simulink model "MARCH_v1_2"  (R2016a)
settings: Solver=FixedStepDiscrete  StartTime=0.0  StopTime=10  FixedStep=.001  RelTol=1e-3
PreLoadFcn:
  | load db.mat
  | initialize_model_param
PostLoadFcn:
  | build_location = fullfile(fileparts(which(bdroot)),'build');
  | 
  | set_param(0, 'CacheFolder', build_location);
  | set_param(0, 'CodeGenFolder', build_location);
InitFcn:
  | % Change dir to model location
  | cd(fileparts(which(bdroot)));
  | 
  | % Run init script
  | init_model;
StartFcn:
  | % Make sure we always move back to model folder
  | cd(fileparts(which(bdroot)));
StopFcn:
  | % Make sure we always move back to model folder
  | cd(fileparts(which(bdroot)));
values from neighbouring files (symbols this model uses):
  n = 1000    [initialize_model_param.m]
undefined symbols (not defined in the file or in its folder): par
libraries: xpcethercatlib x21, slrtlib x5
CloseFcn:
  | % Make sure we always move back to model folder
  | cd(fileparts(which(bdroot)));
  | 
  | set_param(0, 'CacheFolder', '');
  | set_param(0, 'CodeGenFolder', '');
PauseFcn:
  | % Make sure we always move back to model folder
  | cd(fileparts(which(bdroot)));
ContinueFcn:
  | % Make sure we always move back to model folder
  | cd(fileparts(which(bdroot)));
settings Model: SimulationMode=external  Creator=rtheyyun  LastModifiedBy=Projectmarch
settings SolverCC: EnableConcurrentExecution=on  ConcurrentTasks=on
settings DataIOCC: LimitDataPoints=on  SaveFinalState=on  SaveFormat=StructureWithTime  SignalLoggingSaveFormat=ModelDataLogs  InspectSignalLogs=on
settings OptimizationCC: BlockReduction=off  OptimizeBlockIOStorage=off  BufferReuse=off  GlobalBufferReuse=off  ExpressionFolding=off  ExpressionDepthLimit=2147483647  LocalBlockOutputs=off
settings DebuggingCC: ReadBeforeWriteMsg=DisableAll  WriteAfterWriteMsg=DisableAll  WriteAfterReadMsg=DisableAll  UnderspecifiedInitializationDetection=Classic  MergeDetectMultiDrivingBlocksExec=none  SolverPrmCheckMsg=warning  InheritedTsInSrcMsg=none  FcnCallInpInsideContextMsg=UseLocalSettings  AllowSymbolicDim=off  StateNameClashWarn=warning
settings HardwareCC: ProdBitPerPointer=32  ProdLargestAtomicFloat=None  ProdWordSize=32  ProdLongLongMode=on  ProdHWDeviceType=Generic->32-bit x86 compatible
settings ModelReferenceCC: UpdateModelReferenceTargets=Force  PropagateSignalLabelsOutOfModel=off
settings RTWCC: SystemTargetFile=slrt.tlc  TemplateMakefile=slrt_default_tmf  Description=Simulink Real-Time  RTWVerbose=off  RTWCompilerOptimization=on
settings SimulinkRealTimeCC: GeneratePreprocessorConditionals=Disable all  xPCisModelTimeout=off  xPCModelTimeoutSecs=20  xPCConcurrentTasks=on
settings ConfigComp: CovModelRefEnable=Off  CovSFcnEnable=off

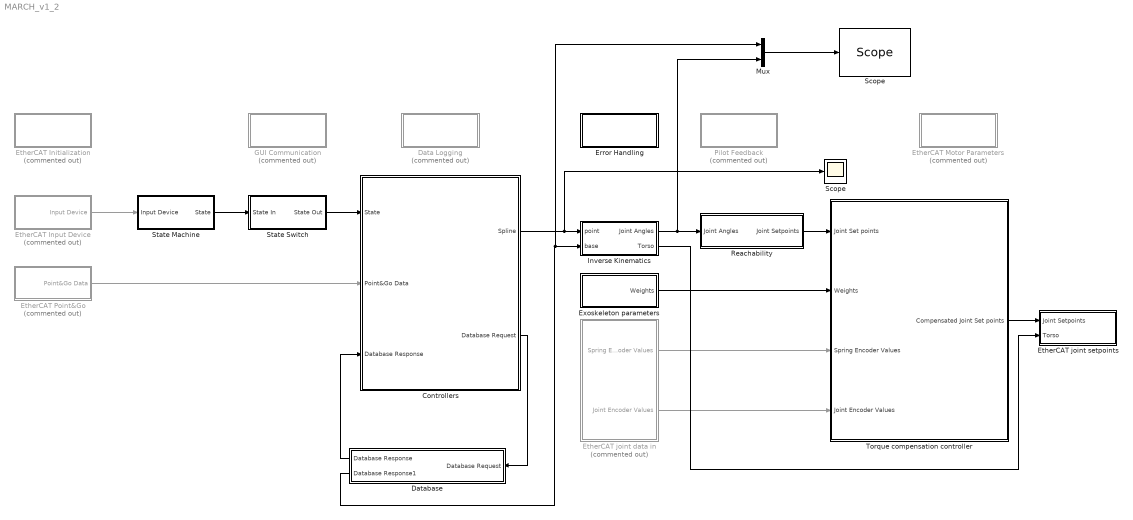
== system MARCH_v1_2 ==
  Controllers : Subsystem
  Data Logging : Subsystem  Commented=on
  Database : Subsystem
  Error Handling : Subsystem
  EtherCAT Initialization : Subsystem  Commented=on
  EtherCAT Input Device : Subsystem  Commented=on
  EtherCAT Motor Parameters : Subsystem  Commented=on
  EtherCAT Point&Go : Subsystem  Commented=on
  EtherCAT joint data in : Subsystem  Commented=on
  EtherCAT joint setpoints : Subsystem
  Exoskeleton parameters : Subsystem
  GUI Communication : Subsystem  Commented=on
  Inverse Kinematics : Subsystem
  Mux : Mux  Inputs=2
  Pilot Feedback : Subsystem  Commented=on
  Reachability : Subsystem
  Scope : Scope
  "Scope " : slrtlib/Displays and Logging/Scope   scopeno=2  scopetype=Target  autostart=on  viewmode=Graphical rolling  formatstr='%15.6f'  grid=on  ylimits=[0,0]  nosamples=25000  noprepostsamples=0  interleave=1  triggermode=FreeRun  triggersignal=1  trigsignalfromport=off  triggerlevel=0.0  triggerslope=Either  triggerscope=1  triggersample=0  filename=data.dat  mode=Lazy  writesize=512  autorestart=off  dynamicfilemode=off  maxwritefilesize=512*1024^2
  State Machine : Subsystem
  State Switch : Subsystem
  Torque compensation controller : Subsystem
  wires:
  Torque compensation controller/1(Compensated Joint Set points) -> EtherCAT joint setpoints/1(Joint Setpoints)
  Reachability/1(Joint Setpoints) -> Torque compensation controller/1(Joint Set points)
  Inverse Kinematics/1(Joint Angles) -> Mux/2, Reachability/1(Joint Angles)
  State Switch/1(State Out) -> Controllers/1(State)
  Controllers/1(Spline) -> Scope/1, Inverse Kinematics/1(point)
  State Machine/1(State) -> State Switch/1(State In)
  Controllers/2(Database Request) -> Database/1(Database Request)
  Database/1(Database Response) -> Controllers/3(Database Response)
  EtherCAT joint data in/1(Spring Encoder Values) -> Torque compensation controller/3(Spring Encoder Values)
  EtherCAT joint data in/2(Joint Encoder Values) -> Torque compensation controller/4(Joint Encoder Values)
  Exoskeleton parameters/1(Weights) -> Torque compensation controller/2(Weights)
  EtherCAT Input Device/1(Input Device) -> State Machine/1(Input Device)
  EtherCAT Point&Go/1(Point&Go Data) -> Controllers/2(Point&Go Data)
  Mux/1 -> "Scope "/1
  Database/2(Database Response1) -> Mux/1, Inverse Kinematics/2(base)
  Inverse Kinematics/2(Torso) -> EtherCAT joint setpoints/2(Torso)

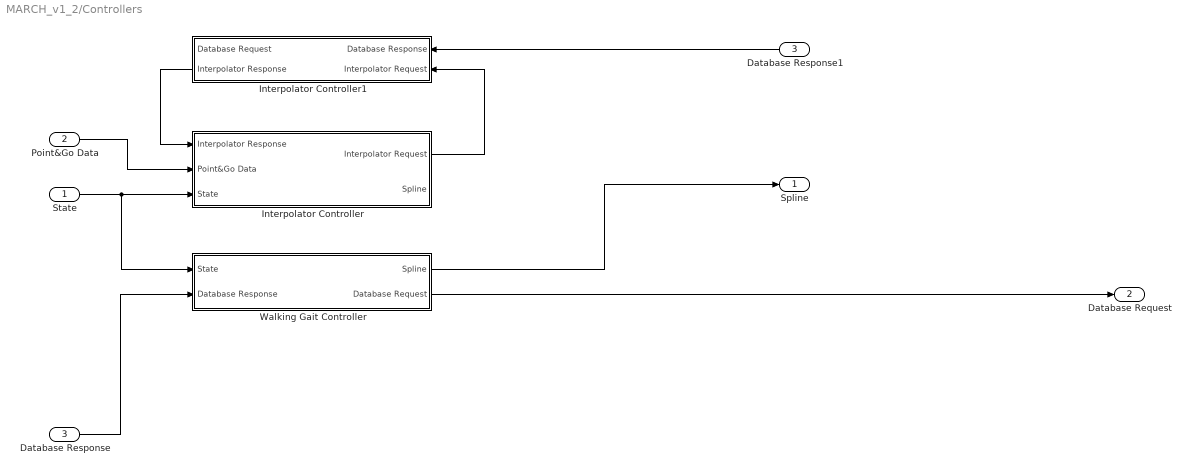
== system MARCH_v1_2/Controllers ==
  State : Inport
  Point&Go Data : Inport  Port=2
  Database Response : Inport  Port=3
  Database Response1 : InportShadow  Port=3
  Interpolator Controller : Subsystem
  Interpolator Controller1 : Subsystem
  Walking Gait Controller : Subsystem
  Spline : Outport
  Database Request : Outport  Port=2
  wires:
  State/1 -> Interpolator Controller/3(State), Walking Gait Controller/1(State)
  Database Response/1 -> Walking Gait Controller/2(Database Response)
  Interpolator Controller/1(Interpolator Request) -> Interpolator Controller1/2(Interpolator Request)
  Interpolator Controller1/2(Interpolator Response) -> Interpolator Controller/1(Interpolator Response)
  Database Response1/1 -> Interpolator Controller1/1(Database Response)
  Walking Gait Controller/2(Database Request) -> Database Request/1
  Walking Gait Controller/1(Spline) -> Spline/1
  Point&Go Data/1 -> Interpolator Controller/2(Point&Go Data)

== system MARCH_v1_2/Data Logging ==

== system MARCH_v1_2/Database ==
  Database Request : Inport
  Database Interface : MATLAB Function  TreatAsAtomicUnit=on
  Database Response : Outport
  Database Response1 : Outport  Port=2
  wires:
  Database Request/1 -> Database Interface/1(request)
  Database Interface/1(spline) -> Database Response/1
  Database Interface/2(swing) -> Database Response1/1

== system MARCH_v1_2/Error Handling ==

== system MARCH_v1_2/EtherCAT Initialization ==
  "EtherCAT Init " : xpcethercatlib/EtherCAT Init   Priority=0  config_file=D:\Software\MATLAB\simulink-models\EtherCAT Config files\quad_slave_both_legs_v1.0.xml  device_id=0  pci_bus=2  pci_slot=0  dctuning=0  enaDebug=off  enaDC=on  errLink=off  masterDbg=off  stateChgDbg=off  baseClock=off  masterCfg=off  logFile='c:\dbglog.txt'  sample_time=0.001000
  Terminator : Terminator
  wires:
  "EtherCAT Init "/1 -> Terminator/1

== system MARCH_v1_2/EtherCAT Input Device ==
  EtherCAT PDO Receive : xpcethercatlib/EtherCAT PDO Receive  Priority=2  sig_name=LHFE.Inputs.jointAngle  sig_offset=208  sig_type=uint32  type_size=32  sig_dim=1  device_id=0  sample_time=0.001000
  Input Device : Outport
  wires:
  EtherCAT PDO Receive/1 -> Input Device/1

== system MARCH_v1_2/EtherCAT Motor Parameters ==

== system MARCH_v1_2/EtherCAT Point&Go ==
  EtherCAT PDO Receive : xpcethercatlib/EtherCAT PDO Receive  Priority=2  sig_name=LHFE.Inputs.jointAngle  sig_offset=208  sig_type=uint32  type_size=32  sig_dim=1  device_id=0  sample_time=0.001000
  Point&Go Data : Outport
  wires:
  EtherCAT PDO Receive/1 -> Point&Go Data/1

== system MARCH_v1_2/EtherCAT joint data in ==
  Joint Encoder EtherCAT : Subsystem
  Spring Encoder EtherCAT : Subsystem  Commented=on
  Spring Encoder Values : Outport
  Joint Encoder Values : Outport  Port=2
  wires:
  Spring Encoder EtherCAT/1(Spring Encoder Values) -> Spring Encoder Values/1
  Joint Encoder EtherCAT/1(Joint Encoder Values) -> Joint Encoder Values/1

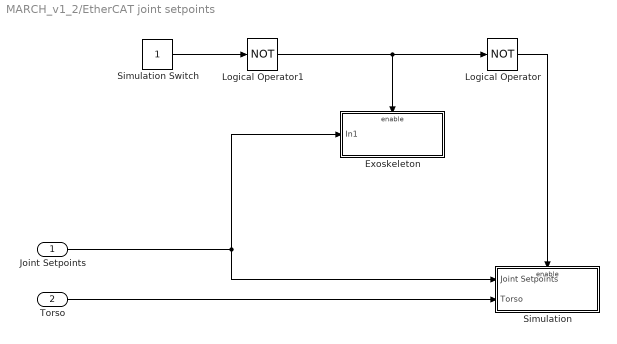
== system MARCH_v1_2/EtherCAT joint setpoints ==
  Joint Setpoints : Inport
  Torso : Inport  Port=2
  Exoskeleton : Subsystem  TreatAsAtomicUnit=on
  Logical Operator : Logic  Operator=NOT  AllPortsSameDT=off  OutDataTypeStr=boolean
  Logical Operator1 : Logic  Operator=NOT  AllPortsSameDT=off  OutDataTypeStr=boolean
  Simulation : Subsystem  TreatAsAtomicUnit=on
  Simulation Switch : Constant
  wires:
  Joint Setpoints/1 -> Exoskeleton/1(In1), Simulation/1(Joint Setpoints)
  Logical Operator1/1 -> Logical Operator/1, Exoskeleton/Enable
  Logical Operator/1 -> Simulation/Enable
  Simulation Switch/1 -> Logical Operator1/1
  Torso/1 -> Simulation/2(Torso)

== system MARCH_v1_2/Exoskeleton parameters ==
  Weights : Outport

== system MARCH_v1_2/GUI Communication ==

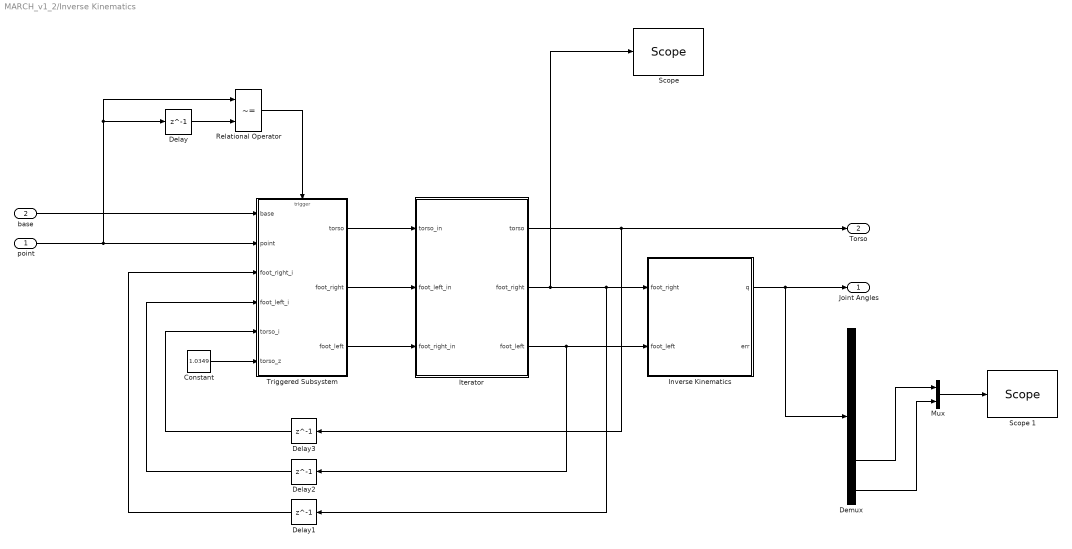
== system MARCH_v1_2/Inverse Kinematics ==
  point : Inport
  base : Inport  Port=2
  Constant : Constant  Value=1.0349
  Delay : Delay  DelayLength=1
  Delay1 : Delay  DelayLength=1  InitialCondition=[0.2073 -0.2467 -1.0349]
  Delay2 : Delay  DelayLength=1  InitialCondition=[0.2073 0.2467 -1.0349]
  Delay3 : Delay  DelayLength=1
  Demux : Demux  Outputs=6
  Inverse Kinematics : MATLAB Function  TreatAsAtomicUnit=on
  Iterator : MATLAB Function  TreatAsAtomicUnit=on
  Mux : Mux  Inputs=2
  Relational Operator : RelationalOperator  Operator=~=  OutDataTypeStr=boolean
  "Scope " : slrtlib/Displays and Logging/Scope   scopeno=1  scopetype=Target  autostart=on  viewmode=Numerical  formatstr='%15.6f'  grid=on  ylimits=[0,0]  nosamples=3  noprepostsamples=0  interleave=1  triggermode=FreeRun  triggersignal=1  trigsignalfromport=off  triggerlevel=0.0  triggerslope=Either  triggerscope=1  triggersample=0  filename=data.dat  mode=Lazy  writesize=512  autorestart=off  dynamicfilemode=off  maxwritefilesize=512*1024^2
  Scope 1 : slrtlib/Displays and Logging/Scope   scopeno=4  scopetype=Target  autostart=on  viewmode=Graphical sliding  formatstr='%15.6f'  grid=on  ylimits=[0,0]  nosamples=100  noprepostsamples=0  interleave=1  triggermode=FreeRun  triggersignal=1  trigsignalfromport=off  triggerlevel=0.0  triggerslope=Either  triggerscope=1  triggersample=0  filename=data.dat  mode=Lazy  writesize=512  autorestart=off  dynamicfilemode=off  maxwritefilesize=512*1024^2
  Triggered Subsystem : Subsystem  TreatAsAtomicUnit=on
  Joint Angles : Outport
  Torso : Outport  Port=2
  wires:
  Inverse Kinematics/1(q) -> Demux/1, Joint Angles/1
  Constant/1 -> Triggered Subsystem/6(torso_z)
  base/1 -> Triggered Subsystem/1(base)
  point/1 -> Relational Operator/1, Delay/1, Triggered Subsystem/2(point)
  Delay/1 -> Relational Operator/2
  Relational Operator/1 -> Triggered Subsystem/Trigger
  Triggered Subsystem/2(foot_right) -> Iterator/2(foot_left_in)
  Delay1/1 -> Triggered Subsystem/3(foot_right_i)
  Delay2/1 -> Triggered Subsystem/4(foot_left_i)
  Delay3/1 -> Triggered Subsystem/5(torso_i)
  Triggered Subsystem/1(torso) -> Iterator/1(torso_in)
  Iterator/1(torso) -> Delay3/1, Torso/1
  Iterator/2(foot_right) -> "Scope "/1, Delay1/1, Inverse Kinematics/1(foot_right)
  Iterator/3(foot_left) -> Delay2/1, Inverse Kinematics/2(foot_left)
  Mux/1 -> Scope 1/1
  Demux/5 -> Mux/1
  Demux/6 -> Mux/2
  Triggered Subsystem/3(foot_left) -> Iterator/3(foot_right_in)

== system MARCH_v1_2/Pilot Feedback ==

== system MARCH_v1_2/Reachability ==
  Joint Angles : Inport
  MATLAB Function : MATLAB Function  TreatAsAtomicUnit=on
  Joint Setpoints : Outport
  wires:
  Joint Angles/1 -> MATLAB Function/1(q)
  MATLAB Function/1(q_out) -> Joint Setpoints/1

== system MARCH_v1_2/State Machine ==
  Input Device : Inport
  Constant : Constant
  State : Outport
  wires:
  Constant/1 -> State/1

== system MARCH_v1_2/State Switch ==
  State In : Inport
  State Out : Outport
  wires:
  State In/1 -> State Out/1

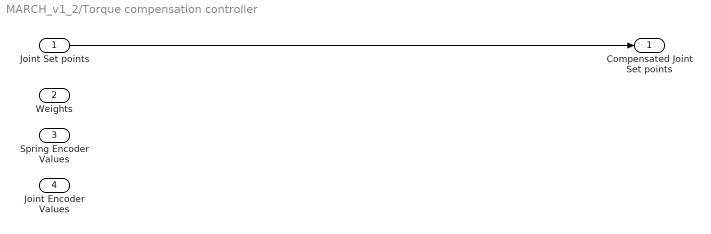
== system MARCH_v1_2/Torque compensation controller ==
  Joint Set points : Inport
  Weights : Inport  Port=2
  Spring Encoder Values : Inport  Port=3
  Joint Encoder Values : Inport  Port=4
  Compensated Joint Set points : Outport
  wires:
  Joint Set points/1 -> Compensated Joint Set points/1

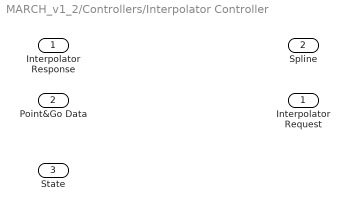
== system MARCH_v1_2/Controllers/Interpolator Controller ==
  Interpolator Response : Inport
  Point&Go Data : Inport  Port=2
  State : Inport  Port=3
  Interpolator Request : Outport
  Spline : Outport  Port=2

== system MARCH_v1_2/Controllers/Interpolator Controller1 ==
  Database Response : Inport
  Interpolator Request : Inport  Port=2
  Database Request : Outport
  Interpolator Response : Outport  Port=2

== system MARCH_v1_2/Controllers/Walking Gait Controller ==
  State : Inport
  Database Response : Inport  Port=2
  Spline : Outport
  Database Request : Outport  Port=2
  wires:
  State/1 -> Database Request/1
  Database Response/1 -> Spline/1

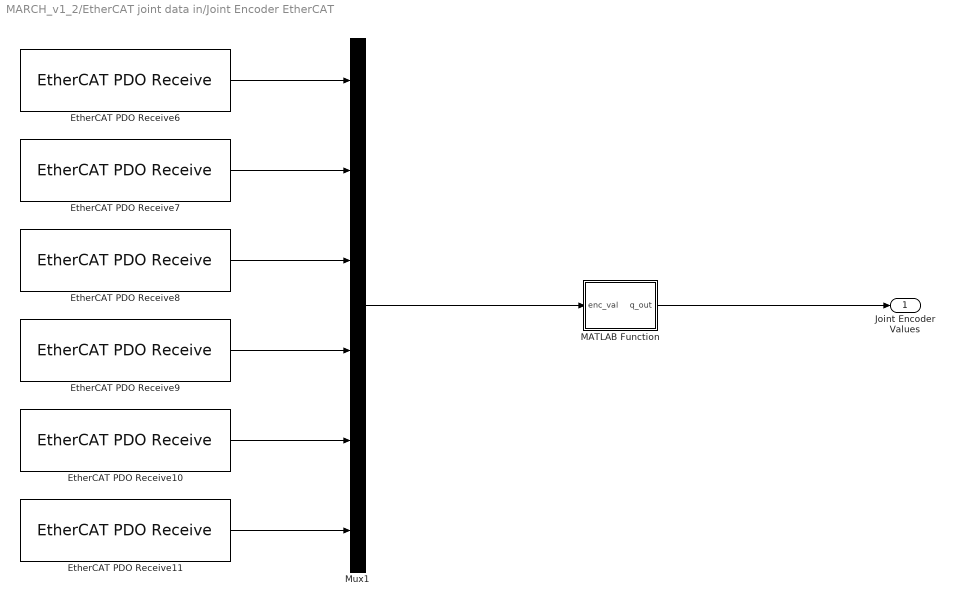
== system MARCH_v1_2/EtherCAT joint data in/Joint Encoder EtherCAT ==
  EtherCAT PDO Receive{6..11} (6 alike) : xpcethercatlib/EtherCAT PDO Receive  Priority=2  sig_name=LHFE.Inputs.jointAngle  sig_offset=208  sig_type=uint32  type_size=32  sig_dim=1  device_id=0  sample_time=0.001000
  MATLAB Function : MATLAB Function  TreatAsAtomicUnit=on
  Mux1 : Mux  Inputs=6
  Joint Encoder Values : Outport
  wires:
  EtherCAT PDO Receive8/1 -> Mux1/3
  EtherCAT PDO Receive9/1 -> Mux1/4
  EtherCAT PDO Receive7/1 -> Mux1/2
  EtherCAT PDO Receive6/1 -> Mux1/1
  EtherCAT PDO Receive10/1 -> Mux1/5
  EtherCAT PDO Receive11/1 -> Mux1/6
  Mux1/1 -> MATLAB Function/1(enc_val)
  MATLAB Function/1(q_out) -> Joint Encoder Values/1

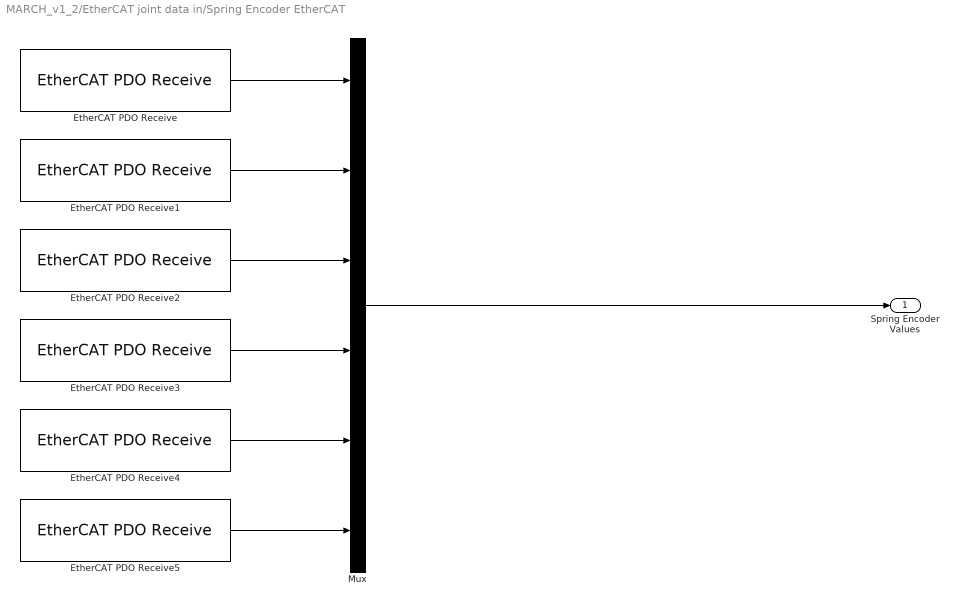
== system MARCH_v1_2/EtherCAT joint data in/Spring Encoder EtherCAT ==
  EtherCAT PDO Receive{,1..5} (6 alike) : xpcethercatlib/EtherCAT PDO Receive  Priority=2  sig_name=LHFE.Inputs.jointAngle  sig_offset=208  sig_type=uint32  type_size=32  sig_dim=1  device_id=0  sample_time=0.001000
  Mux : Mux  Inputs=6
  Spring Encoder Values : Outport
  wires:
  EtherCAT PDO Receive2/1 -> Mux/3
  EtherCAT PDO Receive4/1 -> Mux/5
  Mux/1 -> Spring Encoder Values/1
  EtherCAT PDO Receive5/1 -> Mux/6
  EtherCAT PDO Receive1/1 -> Mux/2
  EtherCAT PDO Receive/1 -> Mux/1
  EtherCAT PDO Receive3/1 -> Mux/4

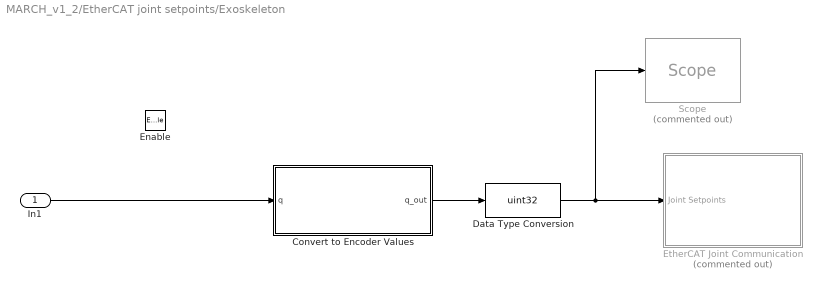
== system MARCH_v1_2/EtherCAT joint setpoints/Exoskeleton ==
  In1 : Inport
  Enable : EnablePort
  Convert to Encoder Values : MATLAB Function  TreatAsAtomicUnit=on
  Data Type Conversion : DataTypeConversion  OutDataTypeStr=uint32
  EtherCAT Joint Communication : Subsystem  Commented=on
  "Scope " : slrtlib/Displays and Logging/Scope   Commented=on  scopeno=2  scopetype=Target  autostart=on  viewmode=Graphical rolling  formatstr='%15.6f'  grid=on  ylimits=[0,0]  nosamples=25000  noprepostsamples=3  interleave=1  triggermode=FreeRun  triggersignal=1  trigsignalfromport=off  triggerlevel=0.0  triggerslope=Either  triggerscope=1  triggersample=0  filename=data.dat  mode=Lazy  writesize=512  autorestart=off  dynamicfilemode=off  maxwritefilesize=512*1024^2
  wires:
  Convert to Encoder Values/1(q_out) -> Data Type Conversion/1
  Data Type Conversion/1 -> "Scope "/1, EtherCAT Joint Communication/1(Joint Setpoints)
  In1/1 -> Convert to Encoder Values/1(q)

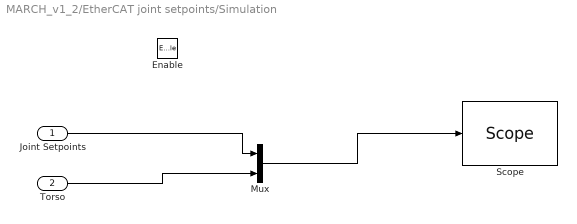
== system MARCH_v1_2/EtherCAT joint setpoints/Simulation ==
  Joint Setpoints : Inport
  Torso : Inport  Port=2
  Enable : EnablePort
  Mux : Mux  Inputs=2
  "Scope " : slrtlib/Displays and Logging/Scope   scopeno=3  scopetype=File  autostart=on  viewmode=Graphical redraw  formatstr='%15.6f'  grid=on  ylimits=[0,0]  nosamples=100000  noprepostsamples=0  interleave=1  triggermode=FreeRun  triggersignal=1  trigsignalfromport=off  triggerlevel=0.0  triggerslope=Either  triggerscope=1  triggersample=0  filename=data.dat  mode=Lazy  writesize=512  autorestart=off  dynamicfilemode=off  maxwritefilesize=512*1024^2
  wires:
  Joint Setpoints/1 -> Mux/1
  Torso/1 -> Mux/2
  Mux/1 -> "Scope "/1

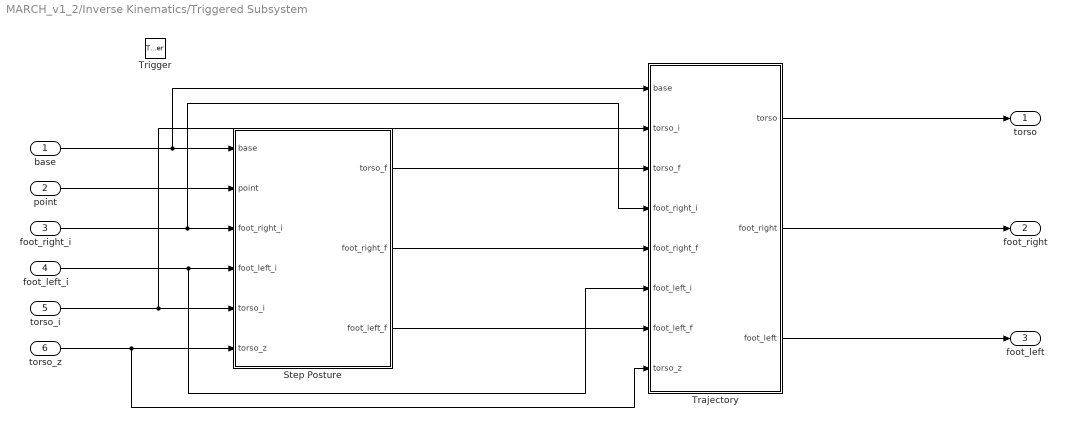
== system MARCH_v1_2/Inverse Kinematics/Triggered Subsystem ==
  base : Inport
  point : Inport  Port=2
  foot_right_i : Inport  Port=3
  foot_left_i : Inport  Port=4
  torso_i : Inport  Port=5
  torso_z : Inport  Port=6
  Trigger : TriggerPort  VariantControl=Variant
  Step Posture : MATLAB Function  TreatAsAtomicUnit=on
  Trajectory : MATLAB Function  TreatAsAtomicUnit=on
  torso : Outport
  foot_right : Outport  Port=2
  foot_left : Outport  Port=3
  wires:
  base/1 -> Trajectory/1(base), Step Posture/1(base)
  torso_z/1 -> Trajectory/8(torso_z), Step Posture/6(torso_z)
  torso_i/1 -> Trajectory/2(torso_i), Step Posture/5(torso_i)
  foot_left_i/1 -> Trajectory/6(foot_left_i), Step Posture/4(foot_left_i)
  foot_right_i/1 -> Trajectory/4(foot_right_i), Step Posture/3(foot_right_i)
  point/1 -> Step Posture/2(point)
  Trajectory/1(torso) -> torso/1
  Trajectory/2(foot_right) -> foot_right/1
  Trajectory/3(foot_left) -> foot_left/1
  Step Posture/1(torso_f) -> Trajectory/3(torso_f)
  Step Posture/2(foot_right_f) -> Trajectory/5(foot_right_f)
  Step Posture/3(foot_left_f) -> Trajectory/7(foot_left_f)

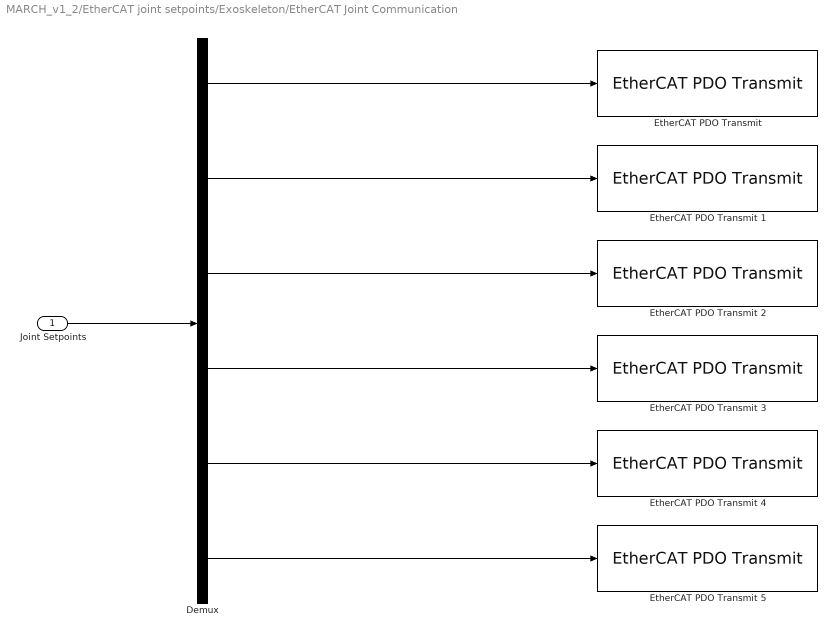
== system MARCH_v1_2/EtherCAT joint setpoints/Exoskeleton/EtherCAT Joint Communication ==
  Joint Setpoints : Inport
  Demux : Demux  Outputs=6
  "EtherCAT PDO Transmit " : xpcethercatlib/EtherCAT PDO Transmit   Priority=3  sig_name=LKFE.Outputs.jointSetpoint  sig_offset=496  sig_type=uint32  type_size=32  sig_dim=1  device_id=0  sample_time=0.001000
  EtherCAT PDO Transmit 1 : xpcethercatlib/EtherCAT PDO Transmit   Priority=3  sig_name=LHFE.Outputs.data0  sig_offset=240  sig_type=uint32  type_size=32  sig_dim=1  device_id=0  sample_time=0.001000
  EtherCAT PDO Transmit 2 : xpcethercatlib/EtherCAT PDO Transmit   Priority=3  sig_name=LHFE.Outputs.data0  sig_offset=240  sig_type=uint32  type_size=32  sig_dim=1  device_id=0  sample_time=0.001000
  EtherCAT PDO Transmit 3 : xpcethercatlib/EtherCAT PDO Transmit   Priority=3  sig_name=LHFE.Outputs.data0  sig_offset=240  sig_type=uint32  type_size=32  sig_dim=1  device_id=0  sample_time=0.001000
  EtherCAT PDO Transmit 4 : xpcethercatlib/EtherCAT PDO Transmit   Priority=3  sig_name=RHFE.Outputs.jointSetpoint  sig_offset=12496  sig_type=uint32  type_size=32  sig_dim=1  device_id=0  sample_time=0.001000
  EtherCAT PDO Transmit 5 : xpcethercatlib/EtherCAT PDO Transmit   Priority=3  sig_name=RKFE.Outputs.jointSetpoint  sig_offset=12784  sig_type=uint32  type_size=32  sig_dim=1  device_id=0  sample_time=0.001000
  wires:
  Demux/5 -> EtherCAT PDO Transmit 4/1
  Demux/6 -> EtherCAT PDO Transmit 5/1
  Demux/4 -> EtherCAT PDO Transmit 3/1
  Demux/1 -> "EtherCAT PDO Transmit "/1
  Demux/3 -> EtherCAT PDO Transmit 2/1
  Demux/2 -> EtherCAT PDO Transmit 1/1
  Joint Setpoints/1 -> Demux/1

== matlab function MARCH_v1_2/Reachability/MATLAB Function ==
  data: q input size=6; q_out output size=6; err output size=6
function [q_out, err] = fcn(q)

joint_limit_min = [-20 -109 -3 -23 -109 -3]'/180*pi;
joint_limit_max = [23 21 121 20 21 121]'/180*pi;

n = size(q,2);
%% Check if all joints are within limits

err = imag(q)~=0 | q<repmat(joint_limit_min,n,1) | q>repmat(joint_limit_max,n,1);
q_out = q;

== matlab function MARCH_v1_2/Inverse Kinematics/Inverse Kinematics ==
  data: foot_right input size=[1 3]; q output size=[1 6]; foot_left input size=[1 3]; par parameter; err output size=[1 6]
function [q,err] = fcn(foot_right, foot_left, par)

[q,err] = inverse_kinematics(foot_right, foot_left, par);

== matlab function MARCH_v1_2/Database/Database Interface ==
  data: request input; spline output size=3; s parameter; swing output size=1
function [spline,swing] = databaseInterface(request, s)
%#codegen
persistent i req base

vector = [0.6647;-0.0805;-1.0349];

if(isempty(i))
   i = zeros(1); 
   vector = [0;0;-1.0349];
end

if(isempty(req))
   req = zeros(1); 
end

if(isempty(base))
   base = zeros(1); 
end

if (req ~= request)
    req = request;
    i = 0;
end

if i < length(s(1).spline)
    i = i+1;
else 
    i = 0;
    if base == 0
        base = 1;
    else 
        base = 0;
    end
end



% if base == 0
%     spline = s(req).spline(:,end);
spline = vector;
% else
%     spline = s(req).spline(:,i);
%    % spline(1,1) = spline(1,1)+s(req).spline(1,end)/2;
% end
swing = base;

== matlab function MARCH_v1_2/Inverse Kinematics/Triggered Subsystem/Step Posture ==
  data: base input size=1; torso_f output size=[1 3]; point input size=[1 3]; foot_right_f output size=[1 3]; foot_right_i input size=[1 3]; foot_left_i input size=[1 3]; torso_i input size=[1 3]; torso_z input size=1; foot_left_f output size=[1 3]; par parameter; n parameter
function [torso_f,foot_right_f,foot_left_f] = step_posture(base,point,foot_right_i,foot_left_i, torso_i, torso_z, par, n)

%% Compute the final x and y positions of torso and feet
if base == 1 %left swing leg
    torso_d = (point+foot_right_i)/2-repmat([par.pelvis_depth 0 0],1,1); %keep torso inbetween stance and swing foot
    foot_right_f = foot_right_i-torso_d; %final right foot position with respect to torso
    foot_left_f = point-torso_d; %final left foot position with respect to torso
else %right swing leg
    torso_d = (point+foot_left_i)/2-repmat([par.pelvis_depth 0 0],1,1); %keep torso inbetween stance and swing foot
    foot_left_f = foot_left_i-torso_d; %final left foot position with respect to torso
    foot_right_f = point-torso_d; %final right foot position with respect to torso
end
torso_f = torso_i+torso_d; %final torso position with respect to world

%% Compute final z positions of torso and feet
% torso height is adapted to keep the stance leg fully stretched
if base == 1 %left swing leg
    torso_f(:,3) = sqrt(torso_z^2+par.pelvis_width^2-(torso_f(:,1)+par.pelvis_depth-torso_i(:,1)-foot_right_i(:,1)).^2-(torso_f(:,2)-par.torso_width-torso_i(:,2)-foot_right_i(:,2)).^2);
else %right swing leg
    torso_f(:,3) = sqrt(torso_z^2+par.pelvis_width^2-(torso_f(:,1)+par.pelvis_depth-torso_i(:,1)-foot_left_i(:,1)).^2-(torso_f(:,2)+par.torso_width-torso_i(:,2)-foot_left_i(:,2)).^2);
end

foot_right_f(:,3) = -torso_f(:,3);
foot_left_f(:,3) = -torso_f(:,3);

== matlab function MARCH_v1_2/EtherCAT joint setpoints/Exoskeleton/Convert to Encoder Values ==
  data: q input; q_out output
function q_out = convertToEncoderValues(q)

persistent RHAA_offset RHFE_offset RKFE_offset LHAA_offset LHFE_offset LKFE_offset
persistent RHAA_scale RHFE_scale RKFE_scale LHAA_scale LHFE_scale LKFE_scale

if (isempty(RHAA_offset))
    RHAA_scale = (391444-360746)/(41/180*pi);
    RHAA_offset = RHAA_scale + 340338;
    
    RHFE_scale = (435150-340338)/(128/180*pi);
    RHFE_offset = RHFE_scale + 340338;
    
    RKFE_scale = (393895-305130)/(121.5/180*pi);
    RKFE_offset = RKFE_scale + 305130;
    
    LHAA_scale = (435150-340338)/(41/180*pi);
    LHAA_offset = LHAA_scale + 340338;
    
    LHFE_scale = (490459-396620)/(128/180*pi);
    LHFE_offset = LHFE_scale + 490469;
    
    LKFE_scale = (458865-369517)/(121.5/180*pi);
    LKFE_offset = LKFE_scale + 458865;
end
% RHAA
% RHFE
% RKFE
% LHAA
% LHFE
% LKFE



% convert joint angles to encoder values
q_out = [(q(1)+22)*RHAA_scale + RHAA_offset;
         (q(2)+18)*RHFE_scale + RHFE_offset;
         (q(3)+120)*RKFE_scale + RKFE_offset;
         LHAA_offset - (q(4)-19)*LHAA_scale;
         LHFE_offset - (q(5)-120)*LHFE_scale;
         LKFE_offset - (q(6)-1.5)*LKFE_scale];

== matlab function MARCH_v1_2/EtherCAT joint data in/Joint Encoder EtherCAT/MATLAB Function ==
  data: enc_val input; q_out output
function q_out = convertToJointAngles(enc_val)

persistent RHAA_in_offset RHFE_in_offset RKFE_in_offset LHAA_in_offset LHFE_in_offset LKFE_in_offset
persistent RHAA_in_scale RHFE_in_scale RKFE_in_scale LHAA_in_scale LHFE_in_scale LKFE_in_scale

if (isempty(RHAA_in_offset))
    RHAA_in_scale = (391444-360746)/(41/180*pi);
    RHAA_in_offset = RHAA_in_scale + 340338;
    
    RHFE_in_scale = (435150-340338)/(128/180*pi);
    RHFE_in_offset = RHFE_in_scale + 340338;
    
    RKFE_in_scale = (393895-305130)/(121.5/180*pi);
    RKFE_in_offset = RKFE_in_scale + 305130;
    
    LHAA_in_scale = (435150-340338)/(41/180*pi);
    LHAA_in_offset = LHAA_in_scale + 340338;
    
    LHFE_in_scale = (490459-396620)/(128/180*pi);
    LHFE_in_offset = LHFE_in_scale + 490469;
    
    LKFE_in_scale = (458865-369517)/(121.5/180*pi);
    LKFE_in_offset = LKFE_in_scale + 458865;
end
% RHAA
% RHFE
% RKFE
% LHAA
% LHFE
% LKFE



% convert joint angles to encoder values
q_out = [(enc_val(1)+22)*RHAA_in_scale + RHAA_in_offset;
         (enc_val(2)+18)*RHFE_in_scale + RHFE_in_offset;
         (enc_val(3)+120)*RKFE_in_scale + RKFE_in_offset;
         LHAA_in_offset - (enc_val(4)-19)*LHAA_in_scale;
         LHFE_in_offset - (enc_val(5)-120)*LHFE_in_scale;
         LKFE_in_offset - (enc_val(6)-1.5)*LKFE_in_scale];

== matlab function MARCH_v1_2/Inverse Kinematics/Triggered Subsystem/Trajectory ==
  data: torso output size=[n 3]; foot_right output size=[n 3]; foot_left output size=[n 3]; base input size=1; torso_i input size=[1 3]; torso_f input size=[1 3]; foot_right_i input size=[1 3]; foot_right_f input size=[1 3]; foot_left_i input size=[1 3]; foot_left_f input size=[1 3]; torso_z input size=1; par parameter; n parameter size=1
function [torso, foot_right, foot_left] = fcn(base,torso_i,torso_f,foot_right_i,foot_right_f,foot_left_i,foot_left_f, torso_z, par, n)

% torso x and y trajectory is a straight line from initial to final position
torso = [linspace(torso_i(:,1),torso_f(:,1),n);linspace(torso_i(:,2),torso_f(:,2),n);zeros(1,n)]';

if base == 1 %left leg is swing leg
    % torso height is adapted to maintain given height
    torso(:,3) = sqrt(torso_z^2+par.pelvis_width^2-(torso(:,1)+par.pelvis_depth-torso_i(:,1)-foot_right_i(:,1)).^2-(torso(:,2)-par.torso_width-torso_i(:,2)-foot_right_i(:,2)).^2);
    
    % right foot is stance foot
    foot_right = repmat(torso_i+foot_right_i,n,1)-torso;
    
    % left foot x and y trajectory is a straight line from initial to final position
    foot_left = [linspace(foot_left_i(:,1),foot_left_f(:,1),n);linspace(foot_left_i(:,2),foot_left_f(:,2),n);zeros(1,n)]';
    
    % left foot z trajectory describes an arc from initial to final foot
    % height. Maximum foot height is determined by parameter foot_height
    midstep = (foot_left_i+torso_i+foot_left_f+torso_f)/2;
    arclength = (midstep-(foot_left_i+torso_i))*(midstep-(foot_left_i+torso_i))';
    radius = (-arclength-par.foot_height^2)/(-2*par.foot_height);
    center = [midstep(1:2) -radius+par.foot_height];
    foot_left(:,3) = sqrt(radius^2-(foot_left(:,1)+torso(1)-center(1)).^2-(foot_left(:,2)+torso(2)-center(2)).^2)+center(3)-torso(3);

else %right leg is swing leg
    % torso height is adapted to maintain given height
    torso(:,3) = sqrt(torso_z^2+par.pelvis_width^2-(torso(:,1)+par.pelvis_depth-torso_i(:,1)-foot_left_i(:,1)).^2-(torso(:,2)+par.torso_width-torso_i(:,2)-foot_left_i(:,2)).^2);
    
    % left foot is stance foot
    foot_left = repmat(torso_i+foot_left_i,n,1)-torso;
    
    % right foot x and y trajectory is a straight line from initial to final position
    foot_right = [linspace(foot_right_i(:,1),foot_right_f(:,1),n);linspace(foot_right_i(:,2),foot_right_f(:,2),n);zeros(1,n)]';
    
    % right foot z trajectory describes an arc from initial to final foot
    % height. Maximum foot height is determined by parameter foot_height
    midstep = (foot_right_i+torso_i+foot_right_f+torso_f)/2;
    arclength = (midstep-(foot_right_i+torso_i))*(midstep-(foot_right_i+torso_i))';
    radius = (-arclength-par.foot_height^2)/(-2*par.foot_height);
    center = [midstep(1:2) -radius+par.foot_height];
    foot_right(:,3) = sqrt(radius^2-(foot_right(:,1)+torso(:,1)-center(1)).^2-(foot_right(:,2)+torso(:,2)-center(2)).^2)+center(3)-torso(:,3);
end

== matlab function MARCH_v1_2/Inverse Kinematics/Iterator ==
  data: torso_in input size=[n 3]; torso output size=[1 3]; foot_right output size=[1 3]; n parameter; foot_left output size=[1 3]; foot_left_in input size=[n 3]; foot_right_in input size=[n 3]
function [torso, foot_right, foot_left] = fcn(torso_in, n, foot_left_in, foot_right_in)
%#codegen
persistent i
if (isempty(i))
    i = 1;
end

torso = torso_in(i,:);
foot_right = foot_right_in(i,:);
foot_left = foot_left_in(i,:);

if i < n-1
    i = i+1;
else

end
